simulink model "sf_simulink"  (R2020a)
settings: Solver=FixedStepAuto  StartTime=0.0  StopTime=10.0  RelTol=1e-3
settings Model: Creator=노호진  LastModifiedBy=노호진
settings OptimizationCC: DefaultParameterBehavior=Inlined  EnhancedBackFolding=on  PassReuseOutputArgsAs=Individual arguments  OptimizeBlockOrder=speed  DifferentSizesBufferReuse=on  OptimizationCustomize=off  EfficientTunableParamExpr=on
settings DebuggingCC: ParameterTunabilityLossMsg=error
settings HardwareCC: ProdBitPerLong=64  ProdHWDeviceType=Intel->x86-64 (Linux 64)  TargetBitPerPointer=64  TargetBitPerSizeT=64  TargetBitPerPtrDiffT=64  TargetLongLongMode=on  TargetIntDivRoundTo=Zero  TargetEndianess=LittleEndian  TargetWordSize=64  TargetHWDeviceType=MATLAB Host  ProdEqTarget=off
settings ModelReferenceCC: EnableRefExpFcnMdlSchedulingChecks=off
settings SFSimCC: SimParseCustomCode=off  SimGenImportedTypeDefs=on  MATLABDynamicMemAlloc=off
settings RTWCC: SystemTargetFile=ert.tlc  GenCodeOnly=on  TemplateMakefile=ert_default_tmf  GenerateReport=on  RTWUseSimCustomCode=on  Toolchain=GNU Tools for ARM Embedded Processors  LaunchReport=on
settings CodeAppCC: ForceParamTrailComments=on  IgnoreCustomStorageClasses=off  OperatorAnnotations=on  SimulinkDataObjDesc=on  SFDataObjDesc=on  InsertBlockDesc=on
settings ERTTargetCC: TargetLangStandard=C99 (ISO)  MultiInstanceERTCode=on  CodeInterfacePackaging=Reusable function  SupportVariableSizeSignals=on  GenerateAllocFcn=on  InlinedParameterPlacement=NonHierarchical  RootIOFormat=Part of model data structure  ERTCustomFileTemplate=example_file_process.tlc  ConvertIfToSwitch=off  PreserveExternInFcnDecls=off

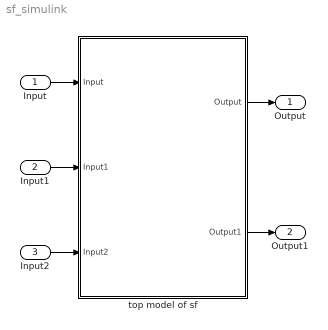
== system sf_simulink ==
  Input : Inport  OutDataTypeStr=Bus:CAM
  Input1 : Inport  Port=2  OutDataTypeStr=Bus: LIDAR
  Input2 : Inport  Port=3  OutDataTypeStr=Bus: CORE
  top model of sf : Subsystem
  Output : Outport  OutDataTypeStr=Bus:OUTPUT
  Output1 : Outport  Port=2  OutDataTypeStr=Bus: MCU_CONTROL
  wires:
  Input/1 -> top model of sf/1(Input)
  Input1/1 -> top model of sf/2(Input1)
  top model of sf/1(Output) -> Output/1
  Input2/1 -> top model of sf/3(Input2)
  top model of sf/2(Output1) -> Output1/1

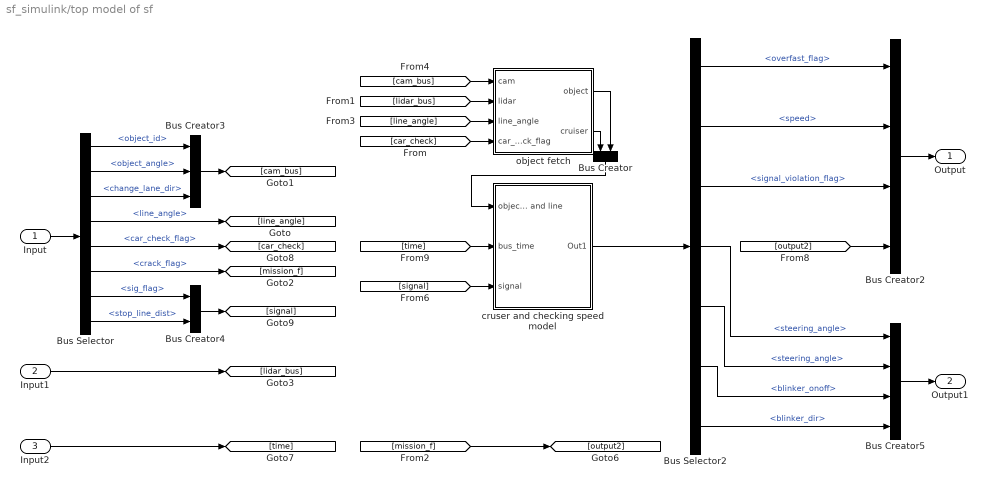
== system sf_simulink/top model of sf ==
  Input : Inport
  Input1 : Inport  Port=2
  Input2 : Inport  Port=3
  Bus Creator : BusCreator  Inputs=2
  Bus Creator2 : BusCreator  Inputs=4
  Bus Creator3 : BusCreator  Inputs=3  OutDataTypeStr=Bus: C_BUS
  Bus Creator4 : BusCreator  Inputs=2
  Bus Creator5 : BusCreator  Inputs=4
  Bus Selector : BusSelector  OutputSignals=object_id,object_angle,change_lane_dir,line_angle,car_check_flag,crack_flag,sig_flag,stop_line_dist
  Bus Selector2 : BusSelector  OutputSignals=overfast_flag,speed,signal_violation_flag,steering_angle,steering_angle,blinker_onoff,blinker_dir
  cruser and checking speed model : Subsystem
  object fetch : Stateflow chart  TreatAsAtomicUnit=on
      settings: PortSchema="{\"entries\":[{\"content\":{\"sides\":[{\"content\":{\"connectorIds\":[\"In1\",\"In2\",\"In3\",\"In4\"]},\"type\":\"ConnectorPlacement.EquallySpacedRectSide\",\"uuid\":\"df99aa18-2a47-4aae-8052-d31a5b92640c\"},{\"content\":{\"connectorIds\":[\"Out2\",\"Out1\"],\"side\":\"RIGHT\"},\"type\":\"ConnectorPlacement.EquallySpacedRectSide\",\"uuid\":\"b65bc204-05f9-4502-ba38-386755187aa6\"},{\"content\":{\"connectorIds\":[],\"side\":\"TOP\"},\"type\":\"ConnectorPlacement.EquallySpacedRectSide\",\"uuid\":\"f13005c3-8b8f-4b1c-aa7b-7f555d22c461\"},{\"content\":{\"connectorIds\":[],\"side\":\"BOTTOM\"},\"type\":\"ConnectorPlacement.EquallySpacedRectSide\",\"uuid\":\"c3f5d7b1-defa-431f-b632-6072e0054c78\"}]},\"type\":\"ConnectorPlacement.EquallySpacedConnector\",\"uuid\":\"0ec5833e-9b22-4c54-b5d3-10ed18be8dad\"}],\"packageUris\":[\"http://schema.mathworks.com/mf0/Connector/19700101\"],\"version\":\"1.0\"}"
  Output : Outport
  Output1 : Outport  Port=2
  wires:
  Input/1 -> Bus Selector/1
  Bus Selector/5 -> [car_check]  "<car_check_flag>"
  Bus Selector/6 -> [mission_f]  "<crack_flag>"
  Input1/1 -> [lidar_bus]
  cruser and checking speed model/1(Out1) -> Bus Selector2/1
  [mission_f] -> [output2]
  Bus Selector2/4 -> Bus Creator5/1  "<steering_angle>"
  Bus Selector2/5 -> Bus Creator5/2  "<steering_angle>"
  Bus Selector2/1 -> Bus Creator2/1  "<overfast_flag>"
  Bus Selector2/2 -> Bus Creator2/2  "<speed>"
  [output2] -> Bus Creator2/4
  Input2/1 -> [time]
  [time] -> cruser and checking speed model/2(bus_time)
  Bus Creator5/1 -> Output1/1
  Bus Creator2/1 -> Output/1
  Bus Selector2/6 -> Bus Creator5/3  "<blinker_onoff>"
  Bus Selector2/7 -> Bus Creator5/4  "<blinker_dir>"
  Bus Selector/1 -> Bus Creator3/1  "<object_id>"
  Bus Selector/2 -> Bus Creator3/2  "<object_angle>"
  Bus Creator3/1 -> [cam_bus]
  Bus Selector/4 -> [line_angle]  "<line_angle>"
  [cam_bus] -> object fetch/1(cam)
  [lidar_bus] -> object fetch/2(lidar)
  object fetch/1(cruiser) -> Bus Creator/1
  Bus Creator/1 -> cruser and checking speed model/1(objects and line)
  [line_angle] -> object fetch/3(line_angle)
  [car_check] -> object fetch/4(car_check_flag)
  Bus Selector/7 -> Bus Creator4/1  "<sig_flag>"
  Bus Selector/8 -> Bus Creator4/2  "<stop_line_dist>"
  Bus Creator4/1 -> [signal]
  [signal] -> cruser and checking speed model/3(signal)
  object fetch/2(object) -> Bus Creator/2
  Bus Selector/3 -> Bus Creator3/3  "<change_lane_dir>"
  Bus Selector2/3 -> Bus Creator2/3  "<signal_violation_flag>"

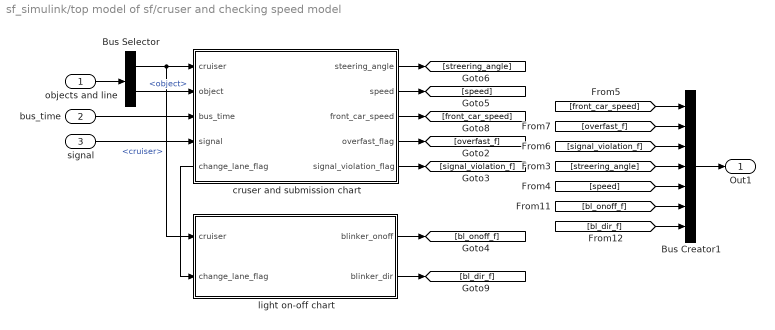
== system sf_simulink/top model of sf/cruser and checking speed model ==
  objects and line : Inport
  bus_time : Inport  Port=2
  signal : Inport  Port=3
  Bus Creator1 : BusCreator  Inputs=7
  Bus Selector : BusSelector  OutputSignals=cruiser,object
  cruser and submission chart : Stateflow chart  TreatAsAtomicUnit=on
      settings: PortSchema="{\"entries\":[{\"content\":{\"sides\":[{\"content\":{\"connectorIds\":[\"In1\",\"In2\",\"In3\",\"In4\",\"Out6\"]},\"type\":\"ConnectorPlacement.EquallySpacedRectSide\",\"uuid\":\"3712cdf8-183b-474a-b0cf-7af3724d8797\"},{\"content\":{\"connectorIds\":[\"Out2\",\"Out3\",\"Out5\",\"Out4\",\"Out1\"],\"side\":\"RIGHT\"},\"type\":\"ConnectorPlacement.EquallySpacedRectSide\",\"uuid\":\"4deee0c1-4fa2-4bc2-92d9-3aa9a84e40af\"},{\"content\":{\"connectorIds\":[],\"side\":\"TOP\"},\"type\":\"ConnectorPlacement.EquallySpacedRectSide\",\"uuid\":\"2883d672-be77-4e9d-ae3e-a181aee2ab46\"},{\"content\":{\"connectorIds\":[],\"side\":\"BOTTOM\"},\"type\":\"ConnectorPlacement.EquallySpacedRectSide\",\"uuid\":\"cd1a3e42-af12-4d84-9b2c-2f0d2a23cd2c\"}]},\"type\":\"ConnectorPlacement.EquallySpacedConnector\",\"uuid\":\"4bc82ee1-d8b8-46d5-8cb4-669cdd6a793c\"}],\"packageUris\":[\"http://schema.mathworks.com/mf0/Connector/19700101\"],\"version\":\"1.0\"}"
  light on-off chart : Stateflow chart  TreatAsAtomicUnit=on
  Out1 : Outport
  wires:
  Bus Creator1/1 -> Out1/1
  [front_car_speed] -> Bus Creator1/1
  [signal_violation_f] -> Bus Creator1/3
  [overfast_f] -> Bus Creator1/2
  cruser and submission chart/4(overfast_flag) -> [overfast_f]
  cruser and submission chart/2(steering_angle) -> [streering_angle]
  cruser and submission chart/3(speed) -> [speed]
  objects and line/1 -> Bus Selector/1
  bus_time/1 -> cruser and submission chart/3(bus_time)
  cruser and submission chart/5(front_car_speed) -> [front_car_speed]
  [streering_angle] -> Bus Creator1/4
  [speed] -> Bus Creator1/5
  light on-off chart/1(blinker_onoff) -> [bl_onoff_f]
  light on-off chart/2(blinker_dir) -> [bl_dir_f]
  [bl_onoff_f] -> Bus Creator1/6
  [bl_dir_f] -> Bus Creator1/7
  signal/1 -> cruser and submission chart/4(signal)
  Bus Selector/1 -> cruser and submission chart/1(cruiser), light on-off chart/1(cruiser)  "<cruiser>"
  Bus Selector/2 -> cruser and submission chart/2(object)  "<object>"
  cruser and submission chart/1(signal_violation_flag) -> [signal_violation_f]
  cruser and submission chart/6(change_lane_flag) -> light on-off chart/2(change_lane_flag)

== stateflow chart sf_simulink/top model of sf/object fetch ==
  state cnt = up_count(cnt, limit) [function]
    (default) -> (junction 136)
    (junction 136) -> (junction 125) [order 1] : [cnt < limit]
        | {cnt = cnt + 1;}
    (junction 131) -> (junction 125)
    (junction 125) -> (junction 133)
    (junction 136) -> (junction 131) [order 2]
  state init
    local_angle_cam = -1;
    local_angle_lidar = -1;
  state running
  (default) -> init
  init -> running
  (junction 99) -> running
  (junction 95) -> (junction 99)
  running -> (junction 180) : /* local data qsort */
      | {
      | local_angle_cam = qsort(cam.object_angle);
      | local_angle_lidar = qsort(lidar.angle);
      | }
  (junction 180) -> (junction 37) : {i = 0; c = 0; l = 0;}
  (junction 227) -> (junction 36) [order 2]
  (junction 36) -> (junction 105) [order 1] : /* each data is bigger than zero,
      | the absolute value of diff between local angles is smaller than three.
      | !!! used data is set minus one !!!
      | data is existed, what... */
      | [
      | local_angle_cam[c] >= 0 && local_angle_lidar[l] >= 0 && ...
      | abs(local_angle_cam[c] - i) < DIFF_ANGLE && ...
      | abs(local_angle_lidar[l] - i) < DIFF_ANGLE && ...
      | (local_angle_cam[c] + local_angle_lidar[l]) / 2 == i
      | ]
  (junction 37) -> (junction 227) [order 1] : [i < 360]
  (junction 227) -> (junction 232) [order 1] : [c >= 10 && l >= 10]
  (junction 36) -> (junction 196) [order 2]
  (junction 105) -> (junction 143) : {
      | each_object.who = 3;
      | each_object.id = search(cam.object_angle, cam.object_id, local_angle_cam[c]);
      | each_object.dist = search(lidar.angle, lidar.dist, local_angle_lidar[l]);
      | object[i] = each_object;
      |
      | c = up_count(c, 10);
      | l = up_count(l, 10);
      | }
  (junction 39) -> (junction 37)
  (junction 37) -> (junction 40) [order 2] : /* data fetch*/
      | {
      | cruiser.line_angle = line_angle;
      | cruiser.car_check_flag = car_check_flag;
      | cruiser.change_lane_dir = cam.change_lane_dir;
      | }
  (junction 196) -> (junction 241) [order 1] : [local_angle_cam[c] < i - DIFF_ANGLE && local_angle_cam[c] >= 0]
      | {c = up_count(c, 10);}
  (junction 196) -> (junction 239) [order 2]
  (junction 241) -> (junction 203)
  (junction 203) -> (junction 239)
  (junction 239) -> (junction 207)
  (junction 207) -> (junction 236) [order 1] : [local_angle_lidar[l] < i - DIFF_ANGLE && local_angle_lidar[l] >= 0]
      | {l = up_count(l, 10);}
  (junction 207) -> (junction 232) [order 2]
  (junction 236) -> (junction 205)
  (junction 205) -> (junction 232)
  (junction 232) -> (junction 38) : {
      | each_object.who = 0;
      | each_object.id = 0;
      | each_object.dist = 0;
      | object[i] = each_object;
      | }
  (junction 40) -> (junction 95)
  (junction 38) -> (junction 39) : {i = i + 1;}
  (junction 143) -> (junction 38)
  data: cnt function_input double; limit function_input double; cnt function_output double; x function_input double size=10; y function_output double size=10; x function_input double size=10; y function_input double size=10; ret function_output double; val function_input double; cam input Bus: C_BUS; lidar input Bus: LIDAR; cruiser output Bus: CRUISER size=1; line_angle input; local_angle_cam local double size=10; local_angle_lidar local double size=10; car_check_flag input; c local int8; l local int8; i local int16; object output Bus: OBJECT size=360; each_object local Bus: OBJECT; DIFF_ANGLE constant double =3
  function y = qsort(x):
    | function y = qsort(x)
    | input = zeros(1,10);
    | for n = 1:10
    |     input(n) = x(n);
    | end
    | input = sort(input);
    | for n = 1:10
    |     y(n) = input(n);
    | end
  function ret = search(x, y, val):
    | function ret = search(x, y, val)
    | ind = find(x == val, 1);
    | ret = y(ind(1));

== stateflow chart sf_simulink/top model of sf/cruser and checking speed model/light on-off chart ==
  state init
    blinker_onoff = 0;
    blinker_dir = 0;
  state running
  (default) -> init
  init -> running
  (junction 32) -> running
  (junction 30) -> (junction 32)
  running -> (junction 17)
  (junction 17) -> (junction 19) [order 1] : /* lane change or not */
      | [change_lane_flag == 1]
  (junction 19) -> (junction 41) [order 1] : [cruiser.change_lane_dir == 1]
  (junction 17) -> (junction 21) [order 2]
  (junction 19) -> (junction 45) [order 2]
  (junction 41) -> (junction 46)
  (junction 21) -> (junction 45) [order 1] : /* turn left */
      | [cruiser.line_angle > ANGLE_STD + 10]
  (junction 21) -> (junction 35) [order 2]
  (junction 45) -> (junction 49) : {blinker_onoff = 1;
      | blinker_dir = 1;}
  (junction 35) -> (junction 46) [order 1] : /* turn right */
      | [cruiser.line_angle < ANGLE_STD - 10]
  (junction 35) -> (junction 28) [order 2] : {blinker_onoff = 0;}
  (junction 46) -> (junction 38) : {blinker_onoff = 1;
      | blinker_dir = 0;}
  (junction 28) -> (junction 30)
  (junction 49) -> (junction 28)
  (junction 38) -> (junction 49)
  data: cruiser input Bus: CRUISER; blinker_onoff output uint8; blinker_dir output uint8; change_lane_flag input; ANGLE_STD constant double =90

== stateflow chart sf_simulink/top model of sf/cruser and checking speed model/cruser and submission chart ==
  state signal_processing [function]
    (default) -> (junction 977)
    (junction 977) -> (junction 965) [order 1] : % yellow or red signal
        | [signal.sig_flag == 1]
    (junction 977) -> (junction 969) [order 2]
    (junction 965) -> (junction 969) [order 2]
    (junction 969) -> (junction 971) : {move_f = 1;}
    (junction 965) -> (junction 970) [order 1] : [signal.stop_line_dist < STOP_DISTANCE]
        | {move_f = 0;}
    (junction 970) -> (junction 971)
    (junction 971) -> (junction 966) : {
        | steering_angle = cruiser.line_angle;
        | save_time = time;
        | time = bus_time.time;
        | }
  state init
    %local
    move_f = 0;
    save_dist = 0;
    save_time = 0;
    time = bus_time.time;
    %output
    steering_angle = cruiser.line_angle;
    speed = 0;
    front_car_speed = 0;
    overfast_flag = 0;
    signal_violation_flag = 0;
    change_lane_flag = 0;
  state normal_running
  state time_reprocessing [function]
    (default) -> (junction 997)
    (junction 997) -> (junction 1001) [order 1] : /* time is mircoseconds.
        | range is 0 ~ 999999*/
        | [time < save_time]
        | {dt = TIME_UNIT - save_time + time;}
    (junction 997) -> (junction 999) [order 2] : {dt = save_time - time;}
    (junction 1001) -> (junction 1003)
    (junction 1003) -> (junction 999)
    (junction 999) -> (junction 1005) : {dt = dt / TIME_UNIT;}
  state check_speeding [function]
    (default) -> (junction 1058)
    (junction 1058) -> (junction 1059) [order 1] : /* overfast checking */
        | [front_car_speed > 60]
        | {overfast_flag = 1;}
    (junction 1058) -> (junction 1064) [order 2]
    (junction 1059) -> (junction 1063)
    (junction 1064) -> (junction 1063) : {overfast_flag = 0;}
  state accelerator [function]
    (default) -> (junction 1024) : {speed += EXTRA_SPEED;}
    (junction 1024) -> (junction 1022) : [speed > 50]
        | {speed = 50;}
  state brake [function]
    (default) -> (junction 1030) : {speed -= EXTRA_SPEED;}
    (junction 1030) -> (junction 1027) : [speed < 0]
        | {speed = 0;}
  state change_lane
  state check_signal_violation [function]
    (default) -> (junction 1127)
    (junction 1127) -> (junction 1129) [order 1] : [signal.sig_flag == 1 && each_obj.dist > (signal.stop_line_dist*100)]
        | {signal_violation_flag = 1;}
    (junction 1127) -> (junction 1139) [order 2] : {signal_violation_flag = 0;}
    (junction 1129) -> (junction 1141)
    (junction 1141) -> (junction 1139)
  (default) -> init
  (junction 599) -> normal_running
  init -> normal_running
  (junction 595) -> (junction 599)
  normal_running -> (junction 562) : {signal_processing();}
  (junction 562) -> (junction 564) [order 2] : /* undiscover the car in front */
  (junction 1123) -> (junction 562) : {change_lane_flag = 0;}
  (junction 1114) -> (junction 1116) : {steering_angle = 110;}
  (junction 564) -> (junction 571)
  (junction 562) -> (junction 1066) [order 1] : /* discover the car in front */
      | [cruiser.car_check_flag == 1 && nonzero_front(object) != 0]
      | {
      | car_num = front_ele(object);
      | save_dist = each_obj.dist;
      | each_obj = object[car_num];
      |
      | check_signal_violation();
      |
      | time_reprocessing();
      | relative_velovity = (each_obj.dist - save_dist) / dt;
      |
      | /* speed unit and relative_velovity unit is centimeters per seconds */
      | front_car_speed = speed + relative_velovity;
      | check_speeding();
      | }
  (junction 1103) -> (junction 1123) [order 2]
  (junction 1112) -> (junction 1114) [order 2]
  (junction 1116) -> (junction 1108)
  (junction 1103) -> (junction 1112) [order 1] : [dt <= 2]
  (junction 1112) -> (junction 1108) [order 1] : [change_lane_dir == 1]
      | {steering_angle = 70;}
  change_lane -> (junction 1103) : {signal_processing();
      | time_reprocessing();}
  (junction 1108) -> (junction 1109)
  (junction 1066) -> change_lane [order 1] : /* the front car is getting closer
      | If the front car is already close, can't change lane */
      | [relative_velovity < 0 && each_obj.dist > 100]
      | {
      | change_lane_dir = cruiser.change_lane_dir;
      | change_lane_flag = 1;
      | speed = 25;
      | }
  (junction 1136) -> change_lane
  (junction 1109) -> (junction 1136) [order 1] : [each_obj.dist > 50]
      | {speed = 25;}
  (junction 1066) -> (junction 575) [order 2]
  (junction 1133) -> (junction 1136)
  (junction 1109) -> (junction 1131) [order 2]
  (junction 571) -> (junction 1012) [order 1] : /* signal light color isn't yellow or red */
      | [signal.sig_flag == 0]
  (junction 1012) -> (junction 1015) : {accelerator();}
  (junction 571) -> (junction 1031) [order 2]
  (junction 1131) -> (junction 1133) : {brake();}
  (junction 1031) -> (junction 1035) [order 1] : /* stop line is close */
      | [signal.stop_line_dist < STOP_DISTANCE]
  (junction 1035) -> (junction 1045)
  (junction 1031) -> (junction 629) [order 2]
  (junction 575) -> (junction 1045) [order 1] : /* the front car is close
      | if it insisted accelerate*/
      | [each_obj.dist < 50]
  (junction 1045) -> (junction 1037) : {brake();}
  (junction 575) -> (junction 1077) [order 2]
  (junction 1015) -> (junction 1037)
  (junction 1037) -> (junction 629)
  (junction 629) -> (junction 1077)
  (junction 1077) -> (junction 595)
  data: x function_input Bus: OBJECT size=360; y function_output double; x function_input Bus: OBJECT size=360; y function_output double; signal_violation_flag output uint8; cruiser input Bus: CRUISER; object input Bus: OBJECT size=360; steering_angle output uint8; speed output uint8; bus_time input Bus: CORE; overfast_flag output uint8; front_car_speed output double; time local double; save_time local double; save_dist local double; signal input Bus: SIGNAL; move_f local double; car_num local double; each_obj local Bus: OBJECT; relative_velovity local double; dt local double; TIME_UNIT constant double =1000000; EXTRA_SPEED constant double =10; STOP_DISTANCE constant double =0.5; change_lane_dir local uint8; change_lane_flag output uint8
  function y = nonzero_front(x):
    | function y = nonzero_front(x)
    | id1 = zeros(1,10);
    | id2 = zeros(1,10);
    | for n = 1:10
    |     id1(n) = x(n).id;
    |     id2(n) = x(n + 350).id;
    | end
    | y = nnz(id1) + nnz(id2);
  function y = front_ele(x):
    | function y = front_ele(x)
    | id = zeros(1,360);
    | for n = 1:360
    |     id(n) = x(n).id;
    | end
    | f1 = find(id(1:10));
    | f2 = find(id(351:360));
    | mn = 0;   mx = 0;
    | if size(f1) > 0
    |     f1 = sort(f1);
    |     mn = min(f1);
    | end
    | if size(f2) > 0
    |     f2 = sort(f2);
    |     mx = max(f2); 
    | end
    | if mn == 0 || mx == 0
    |     if mn ~= 0
    |         y = mn - 1;
    |     else
    |         y = mx - 1;  
    |     end
    | elseif mn > abs(mx - 360)
    |     y = mx - 1;
    | else
    |     y = mn - 1;
    | end
